simulink model "Quarter_car_Model"  (R2018b)
settings: Solver=VariableStepAuto  StartTime=0.0  StopTime=10  RelTol=1e-3
settings Model: Creator=mmf  LastModifiedBy=mmf
settings SolverCC: MaxConsecutiveMinStep=10

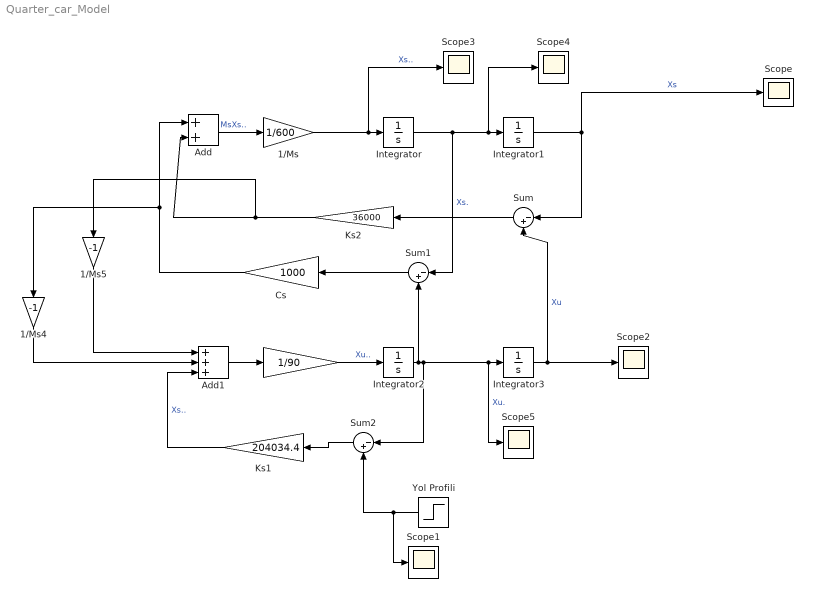
== system Quarter_car_Model ==
  " " : Gain  Gain=1/90
  1/Ms : Gain  Gain=1/600
  1/Ms4 : Gain  Gain=-1
  1/Ms5 : Gain  Gain=-1
  Add : Sum
  Add1 : Sum  Inputs=+++
  Cs : Gain  Gain=1000
  Integrator{,1..3} (4 alike) : Integrator
  Ks1 : Gain  Gain=204034.4
  "Ks2 " : Gain  Gain=36000
  Scope{,1..5} (6 alike) : Scope
  Sum : Sum  Inputs=|-+
  Sum1 : Sum  Inputs=|-+
  Sum2 : Sum  Inputs=|-+
  Yol Profili : Step  SampleTime=0
  wires:
  Integrator3/1 -> Scope2/1, Sum/2  "Xu"
  Integrator/1 -> Sum1/1, Scope4/1, Integrator1/1  "Xs."
  1/Ms/1 -> Scope3/1, Integrator/1  "Xs.."
  Add/1 -> 1/Ms/1  "MsXs.."
  Integrator2/1 -> Sum2/1, Scope5/1, Integrator3/1, Sum1/2  "Xu."
  Add1/1 -> " "/1
  Sum/1 -> "Ks2 "/1
  "Ks2 "/1 -> Add/2, 1/Ms5/1
  " "/1 -> Integrator2/1  "Xu.."
  Sum1/1 -> Cs/1
  Cs/1 -> Add/1, 1/Ms4/1
  1/Ms5/1 -> Add1/1
  1/Ms4/1 -> Add1/2
  Yol Profili/1 -> Scope1/1, Sum2/2
  Sum2/1 -> Ks1/1
  Ks1/1 -> Add1/3  "Xs.."
  Integrator1/1 -> Scope/1, Sum/1  "Xs"
